simulink model "three_phase_pwm_rectifier"  (R2015b)
settings: Solver=FixedStepAuto  SolverMode=SingleTasking  StartTime=0.0  StopTime=10.0  FixedStep=Ts  RelTol=1e-3
values from neighbouring files (symbols this model uses):
  Lline = 1e-3    (= 0.001)    [three_phase_pwm_rectifier.m]
  Rline = 0.01    [three_phase_pwm_rectifier.m]
libraries: powerlib x15, simulink x5, powerlib_meascontrol x5
settings Model: Creator=Eren  LastModifiedBy=Eren

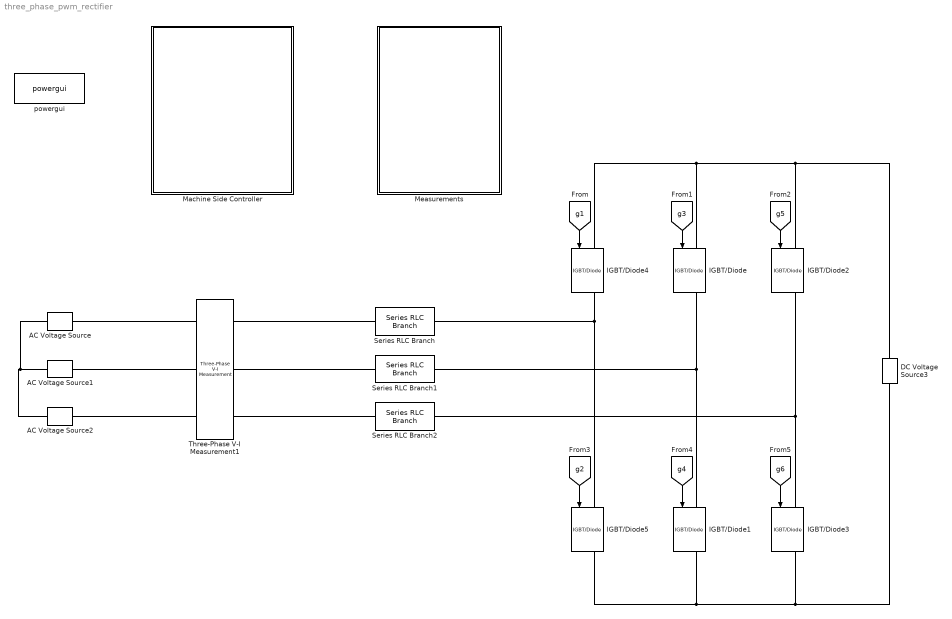
== system three_phase_pwm_rectifier ==
  AC Voltage Source : powerlib/Electrical Sources/AC Voltage Source  Amplitude=400*sqrt(2)  Phase=0  Frequency=50  SampleTime=0  Measurements=None  BusType=swing  Pref=10e3  Qref=0  Qmin=-inf  Qmax=+inf
  AC Voltage Source1 : powerlib/Electrical Sources/AC Voltage Source  Amplitude=400*sqrt(2)  Phase=-120  Frequency=50  SampleTime=0  Measurements=None  BusType=swing  Pref=10e3  Qref=0  Qmin=-inf  Qmax=+inf
  AC Voltage Source2 : powerlib/Electrical Sources/AC Voltage Source  Amplitude=400*sqrt(2)  Phase=120  Frequency=50  SampleTime=0  Measurements=None  BusType=swing  Pref=10e3  Qref=0  Qmin=-inf  Qmax=+inf
  DC Voltage Source3 : powerlib/Electrical Sources/DC Voltage Source  Amplitude=1200  Measurements=None
  IGBT/Diode{,1..5} (6 alike) : powerlib/Power Electronics/IGBT//Diode  Ron=1e-3  Rs=1e5  Cs=inf  Measurements=on
  "Machine Side Controller " : Subsystem
  Measurements : Subsystem
  Series RLC Branch : powerlib/Elements/Series RLC Branch  LConnTagsString=__new0  RConnTagsString=__new0  BranchType=RL  Resistance=Rline  Inductance=Lline  SetiL0=off  InitialCurrent=0  Capacitance=1e-6  Setx0=off  InitialVoltage=0  Measurements=None
  Series RLC Branch1 : powerlib/Elements/Series RLC Branch  LConnTagsString=__new0  RConnTagsString=__new0  BranchType=RL  Resistance=Rline  Inductance=Lline  SetiL0=off  InitialCurrent=0  Capacitance=1e-6  Setx0=off  InitialVoltage=0  Measurements=None
  Series RLC Branch2 : powerlib/Elements/Series RLC Branch  LConnTagsString=__new0  RConnTagsString=__new0  BranchType=RL  Resistance=Rline  Inductance=Lline  SetiL0=off  InitialCurrent=0  Capacitance=1e-6  Setx0=off  InitialVoltage=0  Measurements=None
  Three-Phase V-I Measurement1 : powerlib/Measurements/Three-Phase V-I Measurement  VoltageMeasurement=phase-to-phase  SetLabelV=on  LabelV=Vsabc  Vpu=off  VpuLL=on  CurrentMeasurement=yes  SetLabelI=on  LabelI=Isabc  Ipu=on  Pbase=2.75e6  Vbase=690  OutputType=Complex  PhasorSimulation=off  PSBequivalent=0
  powergui : powerlib/powergui  Priority=2  SimulationMode=Discrete  SolverType=Tustin  SampleTime=10e-6  frequency=60  SPID=off  DisableSnubberDevices=off  DisableRonSwitches=off  DisableVfSwitches=off  SwTol=0  DisplayEquations=off  Interpol=off  ExternalGateDelay=off  methode=off  Ts=0  FunctionMessages=off  echomessages=off  HookPort=off  EnableUseOfTLC=off  x0status=blocks  frequencyindice=0  Pbase=100e6  ErrMax=1e-4  Iterations=50  UnitsV=kV  UnitsW=MW  buscounter=0  RestoreLinks=warning  ResistiveCurrentMeasurement=off  Frange=[0:2:500]  Ylog=off  Xlog=on  ShowGrid=off  save=off  variable=ZData  structure=0  ZoomFFT=on  StartTime=0.0  cycles=1  DisplayStyle=1  fundamental=60  FreqAxis=off  MaxFrequency=1000  frequencyindicesteady=1  RmsSteady=1  display=off
  wires:
  [g1] -> IGBT/Diode4/1
  [g3] -> IGBT/Diode/1
  [g5] -> IGBT/Diode2/1
  [g2] -> IGBT/Diode5/1
  [g4] -> IGBT/Diode1/1
  [g6] -> IGBT/Diode3/1
  connections:
  AC Voltage Source2/LConn1 -- AC Voltage Source/LConn1 -- AC Voltage Source1/LConn1
  Three-Phase V-I Measurement1/RConn1 -- Series RLC Branch/LConn1
  Series RLC Branch1/LConn1 -- Three-Phase V-I Measurement1/RConn2
  Three-Phase V-I Measurement1/LConn3 -- AC Voltage Source2/RConn1
  Three-Phase V-I Measurement1/LConn2 -- AC Voltage Source1/RConn1
  Three-Phase V-I Measurement1/LConn1 -- AC Voltage Source/RConn1
  Series RLC Branch2/LConn1 -- Three-Phase V-I Measurement1/RConn3
  IGBT/Diode5/LConn1 -- Series RLC Branch/RConn1 -- IGBT/Diode4/RConn1
  IGBT/Diode1/LConn1 -- Series RLC Branch1/RConn1 -- IGBT/Diode/RConn1
  IGBT/Diode3/LConn1 -- Series RLC Branch2/RConn1 -- IGBT/Diode2/RConn1
  IGBT/Diode2/LConn1 -- DC Voltage Source3/RConn1 -- IGBT/Diode/LConn1 -- IGBT/Diode4/LConn1
  IGBT/Diode5/RConn1 -- IGBT/Diode1/RConn1 -- IGBT/Diode3/RConn1 -- DC Voltage Source3/LConn1

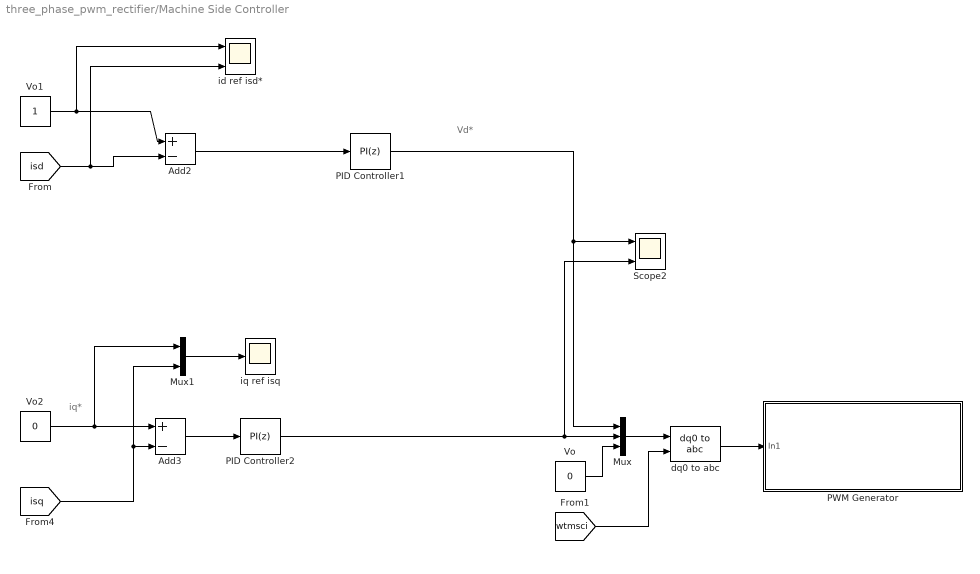
== system three_phase_pwm_rectifier/Machine Side Controller  ==
  note: iq*
  note: Vd*
  Add2 : Sum  Inputs=+-
  Add3 : Sum  Inputs=+-
  Mux : Mux  Inputs=3
  Mux1 : Mux  Inputs=2
  PID Controller1 : simulink/Continuous/PID Controller  Controller=PI  TimeDomain=Discrete-time  SampleTime=-1  IntegratorMethod=Forward Euler  FilterMethod=Forward Euler  Form=Ideal  UseFilter=on  ControllerParametersSource=internal  P=0.05  I=0.1  D=0  N=100  InitialConditionSource=internal  InitialConditionForIntegrator=0  InitialConditionForFilter=0  ExternalReset=none  LimitOutput=on  UpperSaturationLimit=1  LowerSaturationLimit=-1  LinearizeAsGain=on  AntiWindupMode=none  Kb=1  TrackingMode=off  Kt=1  PParamMin=[]  PParamMax=[]  IParamMin=[]  IParamMax=[]  DParamMin=[]  DParamMax=[]  NParamMin=[]  NParamMax=[]  KbParamMin=[]  KbParamMax=[]  KtParamMin=[]  KtParamMax=[]  POutMin=[]  POutMax=[]  IOutMin=[]  IOutMax=[]  DOutMin=[]  DOutMax=[]  NOutMin=[]  NOutMax=[]  KbOutMin=[]  KbOutMax=[]  KtOutMin=[]  KtOutMax=[]  IntegratorOutMin=[]  IntegratorOutMax=[]  FilterOutMin=[]  FilterOutMax=[]  SumOutMin=[]  SumOutMax=[]  SumI1OutMin=[]  SumI1OutMax=[]  SumI2OutMin=[]  SumI2OutMax=[]  SumI3OutMin=[]  SumI3OutMax=[]  SumDOutMin=[]  SumDOutMax=[]  SaturationOutMin=[]  SaturationOutMax=[]  IntegratorContinuousStateAttributes=''  IntegratorStateMustResolveToSignalObject=off  IntegratorRTWStateStorageClass=Auto  FilterContinuousStateAttributes=''  FilterStateMustResolveToSignalObject=off  FilterRTWStateStorageClass=Auto  DifferentiatorICPrevScaledInput=0  DifferentiatorOutMin=[]  DifferentiatorOutMax=[]
  PID Controller2 : simulink/Continuous/PID Controller  Controller=PI  TimeDomain=Discrete-time  SampleTime=-1  IntegratorMethod=Forward Euler  FilterMethod=Forward Euler  Form=Ideal  UseFilter=on  ControllerParametersSource=internal  P=0.07  I=0.1  D=0  N=100  InitialConditionSource=internal  InitialConditionForIntegrator=0  InitialConditionForFilter=0  ExternalReset=none  LimitOutput=on  UpperSaturationLimit=1  LowerSaturationLimit=-1  LinearizeAsGain=on  AntiWindupMode=none  Kb=1  TrackingMode=off  Kt=1  PParamMin=[]  PParamMax=[]  IParamMin=[]  IParamMax=[]  DParamMin=[]  DParamMax=[]  NParamMin=[]  NParamMax=[]  KbParamMin=[]  KbParamMax=[]  KtParamMin=[]  KtParamMax=[]  POutMin=[]  POutMax=[]  IOutMin=[]  IOutMax=[]  DOutMin=[]  DOutMax=[]  NOutMin=[]  NOutMax=[]  KbOutMin=[]  KbOutMax=[]  KtOutMin=[]  KtOutMax=[]  IntegratorOutMin=[]  IntegratorOutMax=[]  FilterOutMin=[]  FilterOutMax=[]  SumOutMin=[]  SumOutMax=[]  SumI1OutMin=[]  SumI1OutMax=[]  SumI2OutMin=[]  SumI2OutMax=[]  SumI3OutMin=[]  SumI3OutMax=[]  SumDOutMin=[]  SumDOutMax=[]  SaturationOutMin=[]  SaturationOutMax=[]  IntegratorContinuousStateAttributes=''  IntegratorStateMustResolveToSignalObject=off  IntegratorRTWStateStorageClass=Auto  FilterContinuousStateAttributes=''  FilterStateMustResolveToSignalObject=off  FilterRTWStateStorageClass=Auto  DifferentiatorICPrevScaledInput=0  DifferentiatorOutMin=[]  DifferentiatorOutMax=[]
  "PWM Generator " : Subsystem
  Scope2 : Scope  NumInputPorts=2
  Vo : Constant  Value=0
  Vo1 : Constant
  Vo2 : Constant  Value=0
  dq0 to abc : powerlib_meascontrol/Transformations/dq0 to abc  Alignment=90 degrees behind phase A axis
  id ref isd* : Scope  NumInputPorts=2
  iq ref isq : Scope
  wires:
  Mux/1 -> dq0 to abc/1
  Vo1/1 -> id ref isd*/1, Add2/1
  Vo/1 -> Mux/3
  [isq] -> Mux1/2, Add3/2
  Add3/1 -> PID Controller2/1
  Add2/1 -> PID Controller1/1
  [isd] -> id ref isd*/2, Add2/2
  Mux1/1 -> iq ref isq/1
  PID Controller1/1 -> Mux/1, Scope2/1
  PID Controller2/1 -> Mux/2, Scope2/2
  Vo2/1 -> Mux1/1, Add3/1
  dq0 to abc/1 -> "PWM Generator "/1(In1)
  [wtmsci] -> dq0 to abc/2

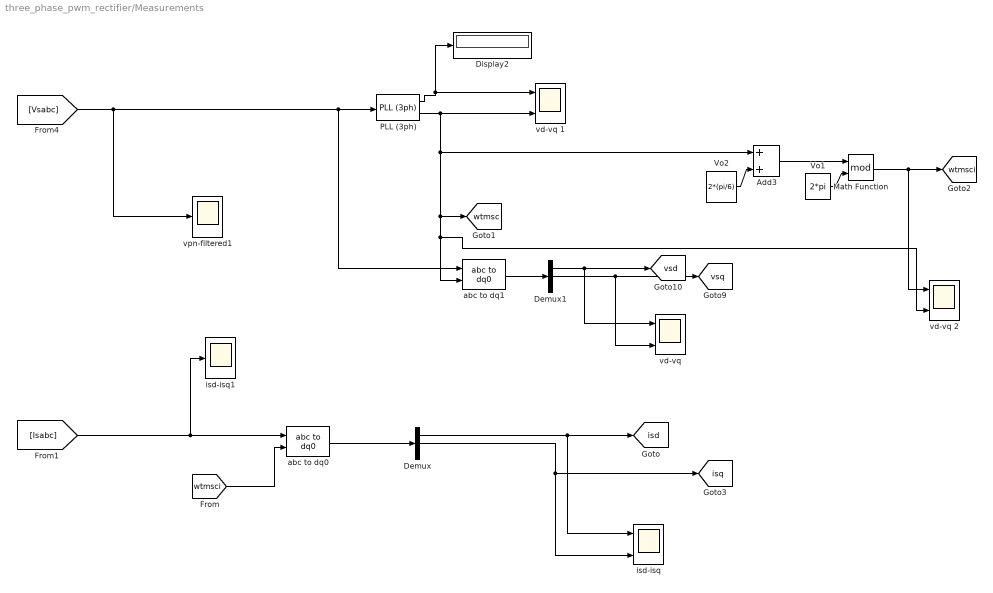
== system three_phase_pwm_rectifier/Measurements ==
  Add3 : Sum
  Demux : Demux  Outputs=3
  Demux1 : Demux  Outputs=3
  Display2 : Display
  Math Function : Math  Operator=mod  SaturateOnIntegerOverflow=on
  PLL (3ph) : powerlib_meascontrol/PLL/PLL (3ph)  Fmin=45  Par_Init=[0, 50]  ParK=[180, 3200, 1]  TcD=1e-4  MaxRateChangeFreq=12  FilterCutOffFreq=25  Ts=0  AGC=on
  Vo1 : Constant  Value=2*pi
  Vo2 : Constant  Value=2*(pi/6)
  abc to dq0 : powerlib_meascontrol/Transformations/abc to dq0  Alignment=90 degrees behind phase A axis
  abc to dq1 : powerlib_meascontrol/Transformations/abc to dq0  Alignment=90 degrees behind phase A axis
  isd-isq : Scope  NumInputPorts=2
  isd-isq1 : Scope
  "vd-vq " : Scope  NumInputPorts=2
  vd-vq 1 : Scope  NumInputPorts=2
  vd-vq 2 : Scope  NumInputPorts=2
  vpn-filtered1 : Scope
  tag scope: isd=global, isq=global, vsd=global, vsq=global, wtmsc=global, wtmsci=global
  wires:
  [Vsabc] -> vpn-filtered1/1, PLL (3ph)/1, abc to dq1/1
  PLL (3ph)/1 -> Display2/1, vd-vq 1/1
  [Isabc] -> isd-isq1/1, abc to dq0/1
  abc to dq0/1 -> Demux/1
  abc to dq1/1 -> Demux1/1
  Demux1/1 -> "vd-vq "/1, [vsd]
  Demux1/2 -> "vd-vq "/2, [vsq]
  Demux/1 -> isd-isq/1, [isd]
  Demux/2 -> [isq], isd-isq/2
  Math Function/1 -> vd-vq 2/1, [wtmsci]
  Add3/1 -> Math Function/1
  Vo2/1 -> Add3/2
  Vo1/1 -> Math Function/2
  [wtmsci] -> abc to dq0/2
  PLL (3ph)/2 -> Add3/1, [wtmsc], vd-vq 2/2, abc to dq1/2, vd-vq 1/2

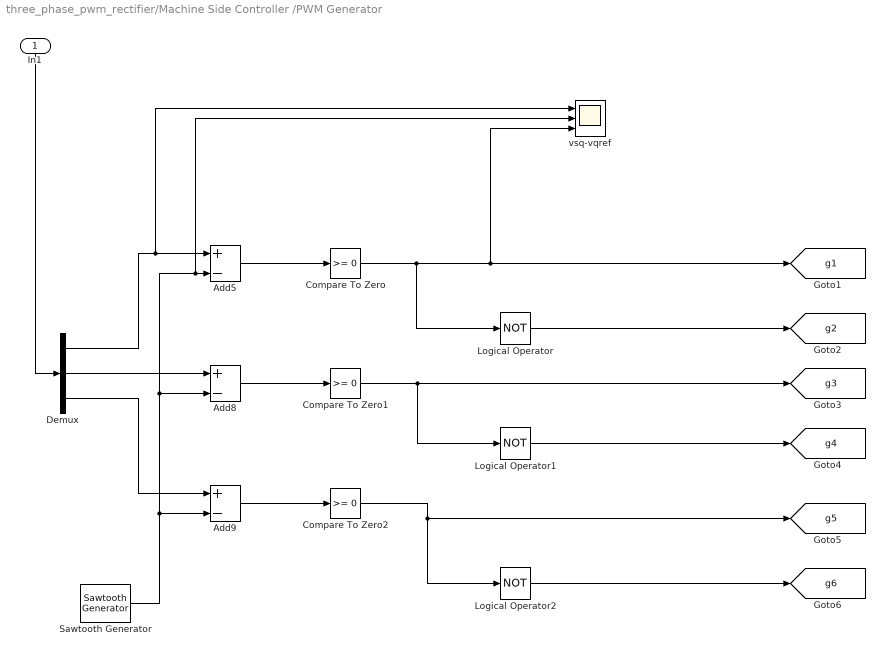
== system three_phase_pwm_rectifier/Machine Side Controller /PWM Generator  ==
  In1 : Inport
  Add5 : Sum  Inputs=+-
  Add8 : Sum  Inputs=+-
  Add9 : Sum  Inputs=+-
  Compare To Zero : simulink/Logic and Bit Operations/Compare To Zero  relop=>=  OutDataTypeStr=boolean
  Compare To Zero1 : simulink/Logic and Bit Operations/Compare To Zero  relop=>=  OutDataTypeStr=boolean
  Compare To Zero2 : simulink/Logic and Bit Operations/Compare To Zero  relop=>=  OutDataTypeStr=boolean
  Demux : Demux  Outputs=3
  Logical Operator : Logic  Operator=NOT  AllPortsSameDT=off  OutDataTypeStr=boolean
  Logical Operator1 : Logic  Operator=NOT  AllPortsSameDT=off  OutDataTypeStr=boolean
  Logical Operator2 : Logic  Operator=NOT  AllPortsSameDT=off  OutDataTypeStr=boolean
  Sawtooth Generator : powerlib_meascontrol/Pulse & Signal Generators/Sawtooth Generator  Freq=drivefreq  Phase=0  Ts=0
  vsq-vqref : Scope  NumInputPorts=3
  tag scope: g1=global, g2=global, g3=global, g4=global, g5=global, g6=global
  wires:
  Add8/1 -> Compare To Zero1/1
  Demux/1 -> vsq-vqref/1, Add5/1
  Compare To Zero/1 -> Logical Operator/1, [g1], vsq-vqref/3
  Add9/1 -> Compare To Zero2/1
  Demux/2 -> Add8/1
  Demux/3 -> Add9/1
  Logical Operator2/1 -> [g6]
  Add5/1 -> Compare To Zero/1
  In1/1 -> Demux/1
  Sawtooth Generator/1 -> Add8/2, vsq-vqref/2, Add5/2, Add9/2
  Compare To Zero1/1 -> [g3], Logical Operator1/1
  Logical Operator/1 -> [g2]
  Compare To Zero2/1 -> Logical Operator2/1, [g5]
  Logical Operator1/1 -> [g4]
